simulink model "super"  (R2014a)
settings: Solver=ode3  SolverMode=SingleTasking  StartTime=0.0  StopTime=24*3600  FixedStep=1  RelTol=1e-3
libraries: refrigeration x6
settings Model: Creator=avenger  LastModifiedBy=avenger
settings SolverCC: AutoInsertRateTranBlk=on
settings DataIOCC: LimitDataPoints=off

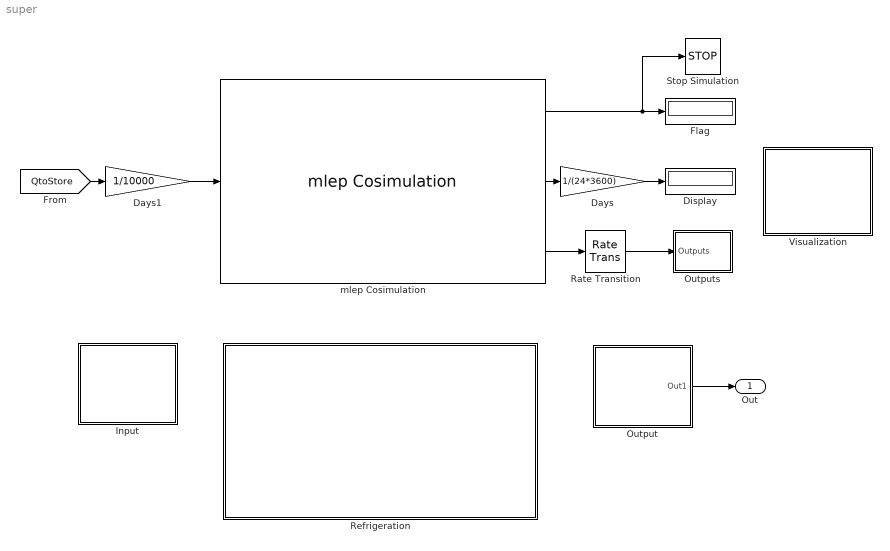
== system super ==
  Days : Gain  Gain=1/(24*3600)
  Days1 : Gain  Gain=1/10000
  Display : Display
  Flag : Display
  Input : Subsystem
  Output : Subsystem
  Outputs : Subsystem
  Rate Transition : RateTransition
  Refrigeration : Subsystem
  Stop Simulation : Stop
  Visualization : Subsystem
  mlep Cosimulation : refrigeration/mlep Cosimulation  progname='runenergyplus'  idf='super_noSi_noCa'  weather='USA_FL_Miami.Intl.AP.722020_TMY3'  timeout=2000  step=300  numinput=1  numoutput=5  bcvtbpath='/home/avenger/Documents/git/mlep_v2.0/MLE+/bcvtb'
  Out : Outport  InitialOutput=0
  wires:
  mlep Cosimulation/2 -> Days/1
  mlep Cosimulation/1 -> Stop Simulation/1, Flag/1
  Days/1 -> Display/1
  mlep Cosimulation/3 -> Rate Transition/1
  [QtoStore] -> Days1/1
  Output/1(Out1) -> Out/1
  Rate Transition/1 -> Outputs/1(Outputs)
  Days1/1 -> mlep Cosimulation/1

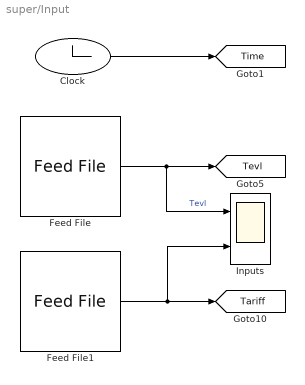
== system super/Input ==
  Clock : Clock
  Feed File : refrigeration/Feed File  filename='input.txt'  timestep=600  feedstep=3600
  Feed File1 : refrigeration/Feed File  filename='tariff.txt'  timestep=300  feedstep=3600
  Inputs : Scope  NumInputPorts=2
      settings: ShowLegends=on  TimeRange=90000  YMin=0~0  YMax=25~0.1  SaveName=ScopeData3  SampleInput=on
  tag scope: Tariff=global, Tevl=global, Time=global
  wires:
  Feed File/1 -> [Tevl], Inputs/1  "Tevl"
  Clock/1 -> [Time]
  Feed File1/1 -> Inputs/2, [Tariff]

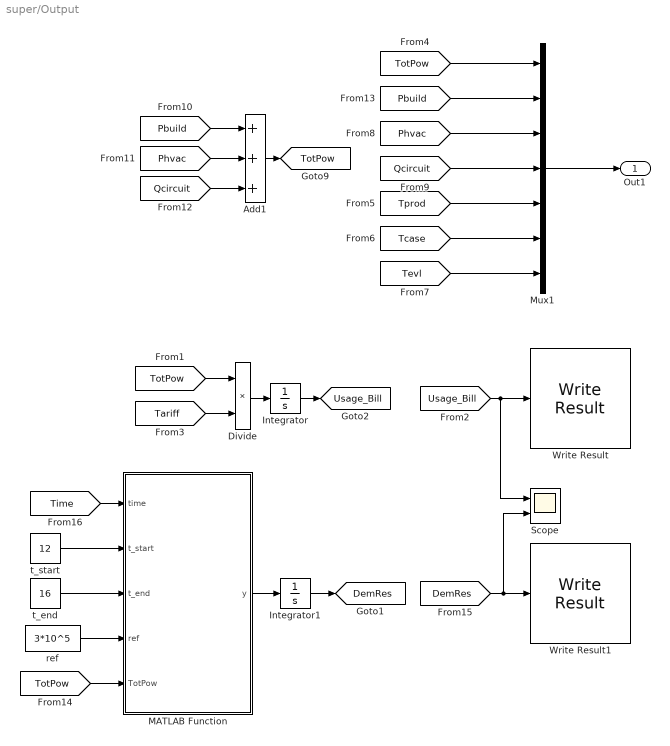
== system super/Output ==
  Add1 : Sum  Inputs=+++
  Divide : Product  Inputs=**
  Integrator : Integrator  UpperSaturationLimit=10^7  LowerSaturationLimit=-10^7
  Integrator1 : Integrator  UpperSaturationLimit=10^7  LowerSaturationLimit=-10^7
  MATLAB Function : MATLAB Function  TreatAsAtomicUnit=on
  Mux1 : Mux  Inputs=7
  Scope : Scope  NumInputPorts=2
      settings: ShowLegends=on  TimeRange=90000  YMin=-500000000~0  YMax=1500000000~1500000000  SaveName=ScopeData2
  Write Result : refrigeration/Write Result  filename='result.txt'  timestep=3600
  Write Result1 : refrigeration/Write Result  filename='result1.txt'  timestep=3600
  ref : Constant  Value=3*10^5
  t_end : Constant  Value=16
  t_start : Constant  Value=12
  Out1 : Outport  InitialOutput=0
  tag scope: DemRes=global, TotPow=global, Usage_Bill=global
  wires:
  [TotPow] -> Divide/1
  [Tariff] -> Divide/2
  Divide/1 -> Integrator/1
  [Pbuild] -> Add1/1
  [Phvac] -> Add1/2
  [Qcircuit] -> Add1/3
  Add1/1 -> [TotPow]
  [Pbuild] -> Mux1/2
  [Tcase] -> Mux1/6
  [Tprod] -> Mux1/5
  [Tevl] -> Mux1/7
  [Phvac] -> Mux1/3
  [Qcircuit] -> Mux1/4
  [TotPow] -> Mux1/1
  Mux1/1 -> Out1/1
  Integrator/1 -> [Usage_Bill]
  [Usage_Bill] -> Scope/1, Write Result/1
  [DemRes] -> Scope/2, Write Result1/1
  [Time] -> MATLAB Function/1(time)
  t_start/1 -> MATLAB Function/2(t_start)
  t_end/1 -> MATLAB Function/3(t_end)
  ref/1 -> MATLAB Function/4(ref)
  [TotPow] -> MATLAB Function/5(TotPow)
  MATLAB Function/1(y) -> Integrator1/1
  Integrator1/1 -> [DemRes]

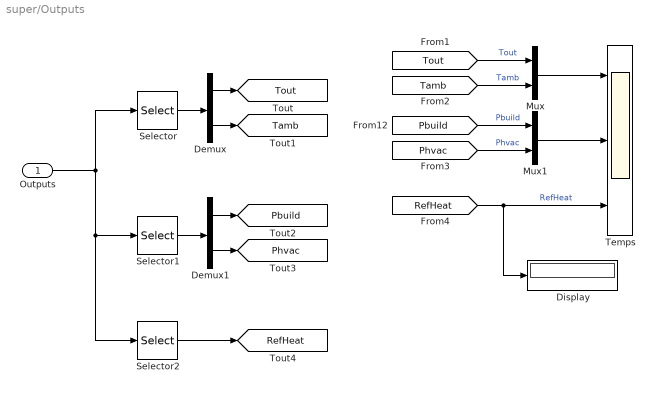
== system super/Outputs ==
  Outputs : Inport
  Demux : Demux  Outputs=2
  Demux1 : Demux  Outputs=2
  Display : Display
  Mux : Mux  Inputs=2
  Mux1 : Mux  Inputs=2
  Selector : Selector  InputPortWidth=5  Indices=[1:2]
  Selector1 : Selector  InputPortWidth=5  Indices=[3:4]
  Selector2 : Selector  InputPortWidth=5  Indices=[5]
  Temps : Scope  NumInputPorts=3
      settings: ShowLegends=on  TimeRange=86400  YMin=0~0~-8000  YMax=32.5~375000~0
  tag scope: Pbuild=global, Phvac=global, RefHeat=global, Tamb=global, Tout=global
  wires:
  [Tout] -> Mux/1  "Tout"
  [Tamb] -> Mux/2  "Tamb"
  Mux/1 -> Temps/1
  [Pbuild] -> Mux1/1  "Pbuild"
  Selector/1 -> Demux/1
  Demux/1 -> [Tout]
  Demux/2 -> [Tamb]
  Selector1/1 -> Demux1/1
  Demux1/1 -> [Pbuild]
  Demux1/2 -> [Phvac]
  Mux1/1 -> Temps/2
  [Phvac] -> Mux1/2  "Phvac"
  Outputs/1 -> Selector2/1, Selector1/1, Selector/1
  Selector2/1 -> [RefHeat]
  [RefHeat] -> Display/1, Temps/3  "RefHeat"

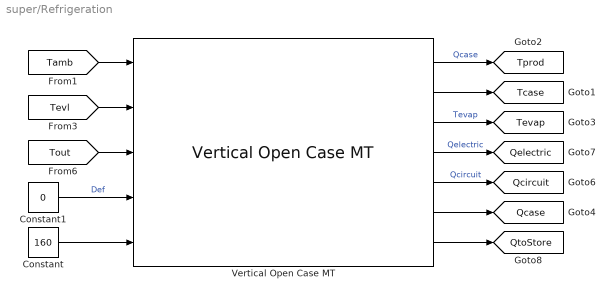
== system super/Refrigeration ==
  Constant : Constant  Value=160
  Constant1 : Constant  Value=0
  Vertical Open Case MT : refrigeration/Vertical Open Case MT  Beta=1.5164e-4  Ccase=2.0114e06  Cprod=9.9574e4  Rce=9.5658e-1  Rac=1.1323e-1  Tprod_0=-20  Tcase_0=-20
  tag scope: Qcase=global, Qcircuit=global, Qelectric=global, QtoStore=global, Tcase=global, Tevap=global, Tprod=global
  wires:
  [Tevl] -> Vertical Open Case MT/2
  Constant/1 -> Vertical Open Case MT/5
  Constant1/1 -> Vertical Open Case MT/4  "Def"
  Vertical Open Case MT/6 -> [Qcase]
  [Tamb] -> Vertical Open Case MT/1
  [Tout] -> Vertical Open Case MT/3
  Vertical Open Case MT/1 -> [Tprod]  "Qcase"
  Vertical Open Case MT/2 -> [Tcase]
  Vertical Open Case MT/3 -> [Tevap]  "Tevap"
  Vertical Open Case MT/4 -> [Qelectric]  "Qelectric"
  Vertical Open Case MT/7 -> [QtoStore]
  Vertical Open Case MT/5 -> [Qcircuit]  "Qcircuit"

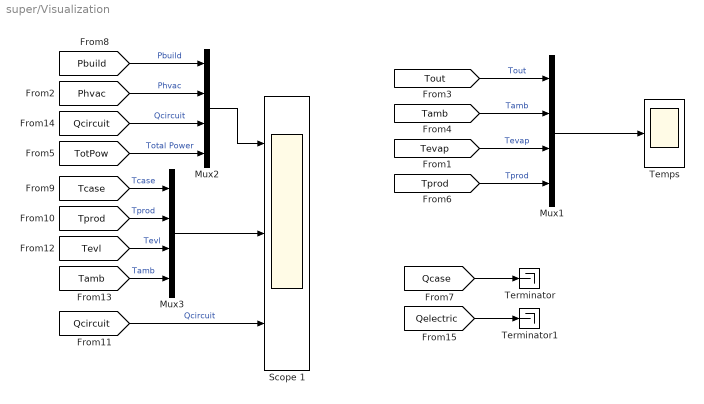
== system super/Visualization ==
  Mux1 : Mux
  Mux2 : Mux
  Mux3 : Mux
  Scope 1 : Scope  NumInputPorts=3
      settings: ShowLegends=on  TimeRange=86400  YMin=-50000~-20~-50000  YMax=950000~22.5~950000  SaveName=ScopeData4
  Temps : Scope
      settings: ShowLegends=on  TimeRange=90000  YMin=-40  YMax=40
  Terminator : Terminator
  Terminator1 : Terminator
  wires:
  Mux1/1 -> Temps/1
  [Tout] -> Mux1/1  "Tout"
  [Tamb] -> Mux1/2  "Tamb"
  [Tevap] -> Mux1/3  "Tevap"
  [Tprod] -> Mux1/4  "Tprod"
  [Pbuild] -> Mux2/1  "Pbuild"
  [Tcase] -> Mux3/1  "Tcase"
  [Tprod] -> Mux3/2  "Tprod"
  [Tevl] -> Mux3/3  "Tevl"
  [Tamb] -> Mux3/4  "Tamb"
  [Qcircuit] -> Mux2/3  "Qcircuit"
  Mux2/1 -> Scope 1/1
  [Qcircuit] -> Scope 1/3  "Qcircuit"
  Mux3/1 -> Scope 1/2
  [Phvac] -> Mux2/2  "Phvac"
  [TotPow] -> Mux2/4  "Total Power"
  [Qcase] -> Terminator/1
  [Qelectric] -> Terminator1/1

== matlab function super/Output/MATLAB Function ==
  data: time input; y output; t_start input; t_end input; ref input; TotPow input
function y = fcn(time,t_start,t_end,ref,TotPow)
%#codegen


if (time > t_start*3600 && time < t_end*3600)
    y = TotPow - ref;
else
    y = 0;
end
